simulink model "Cruise_Model_V8_QRTuning_LQI"  (R2024a)
settings: Solver=ode23t  StartTime=0.0  StopTime=20  RelTol=1e-3
values from neighbouring files (symbols this model uses):
  coefficients =     [UAM2.mat]    (also in VX4_cur.mat; VX4data.mat; alexisignoringme11UAM2.mat; alexisignoringme12.mat)
  Kpi = lqr(sys, Q, R)    [QRerr_LQI.m]    (also in alexisignoringme8.mat = [9.62344892608e-17 -1.21933000029e-16 1.4312558077e-15 29.45)
  mission =     [alexisignoringme.mat]    (also in alexisignoringme11UAM2.mat; alexisignoringme12.mat; alexisignoringme13.mat; alexisignoringme14.mat)
  q = 0.5*1.225*airflow.U^2    [VLMV3.m]    (also in VLMV3_modified.m = 0.5*1.225*airflow.U^2*Sref)
  referenceGeo =     [VX4data.mat]    (also in alexisignoringme.mat; alexisignoringme11UAM2.mat; alexisignoringme12.mat; alexisignoringme13.mat)
  Ue = U(:,idx(2)+1)    [QRerr_LQI.m]    (also in QRerr_p.m; alexisignoringme4.mat = [0.01662518914 6.61806403433e-08 9.21309449136e-07 1460.2523; alexisignoringme5.mat = [0 0 0 0 0 -1471.90874183 1.06985703496e-06 -4.11944256484e-; alexisignoringme6.mat = [0 0 0 0 0 -1471.90874183 1.06985703496e-06 -4.11944256484e-)
  X = [0.00351660116596 0 -9.99999602467 0 0 0 2.75026701025e-08 -4.1982332666e-06 -1.5333765693e-08 0.000503097278932 0 -6.54626389426e-11 ... (630 elements, 9x5x14)]    [alexisignoringme.mat]    (also in alexisignoringme12.mat = [0.000256495736971 0 -9.99999647184 0 0 0 0 -3.73764411116e-; alexisignoringme13.mat = [0.00833666803911 0 -10.0000021435 0 0 0 0 7.14203458163e-06; alexisignoringme14.mat = [0.00833666803911 0 -10.0000021435 0 0 0 0 7.14203458163e-06; alexisignoringme4.mat = [0.00351658839646 0 -9.99999599468 0 0 0 2.7327442949e-09 -4)
  Xe = X(:,idx(2)+1)    [QRerr_LQI.m]    (also in QRerr_p.m; alexisignoringme4.mat = [24.9726490597 0 -1.16896704065 0 0 0 -8.24889531393e-07 -0.; alexisignoringme5.mat = [24.9726490597 0 -1.16896704065 0 0 0 -8.24889531393e-07 0.0; alexisignoringme6.mat = [24.9726490597 0 -1.16896704065 0 0 0 -8.24889531393e-07 0.0)
  Xes = X(:,idx(2))    [QRerr_LQI.m]    (also in QRerr_p.m; alexisignoringme4.mat = [0.00351658839646 0 -9.99999599468 0 0 0 2.7327442949e-09 -4; alexisignoringme5.mat = [0 0 -1.11199998303 0 0 0 -1.38069247376e-09 1.48137256273e-; alexisignoringme6.mat = [0 0 -1.11199998303 0 0 0 -1.38069247376e-09 1.48137256273e-)
undefined symbols (not defined in the file or in its folder): F, Light, MIL
libraries: slpidlib x14, aerolibwind2 x8, aerolibatmos2 x4, shared6dof x1
(part 3 of 3)

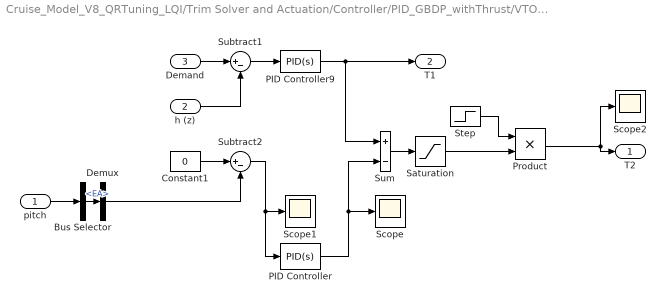
== system Cruise_Model_V8_QRTuning_LQI/Trim Solver and Actuation/Controller/PID_GBDP_withThrust/VTOL Control Path ==
  pitch : Inport
  h (z) : Inport  Port=2
  Demand : Inport  Port=3
  Bus Selector : BusSelector  OutputSignals=EA
  Constant1 : Constant  Value=0
  Demux : Demux  Outputs=3
  PID Controller : slpidlib/PID Controller  Controller=PID  Form=Parallel  TimeDomain=Continuous-time  UseExternalTs=off  SampleTime=-1  IntegratorMethod=Forward Euler  FilterMethod=Forward Euler  ControllerParametersSource=internal  P=2347  I=2604  UseKiTs=off  D=519  UseExternalDerivativeSource=off  N=129  UseFilter=on  TunerSelectOption=Transfer Function Based (PID Tuner App)  InitialConditionSource=internal  InitialConditionForIntegrator=0  InitialConditionForFilter=0  DifferentiatorICPrevScaledInput=0  ExternalReset=none  TrackingMode=off  Kt=1  LimitOutput=on  SatLimitsSource=internal  UpperSaturationLimit=800  LowerSaturationLimit=-800  LinearizeAsGain=on  AntiWindupMode=clamping  Kb=1  LimitIntegrator=off  UpperIntegratorSaturationLimit=inf  LowerIntegratorSaturationLimit=-inf  POutMin=[]  POutMax=[]  IOutMin=[]  IOutMax=[]  DOutMin=[]  DOutMax=[]  NOutMin=[]  NOutMax=[]  SumOutMin=[]  SumOutMax=[]  SaturationOutMin=[]  SaturationOutMax=[]  PParamMin=[]  PParamMax=[]  IParamMin=[]  IParamMax=[]  DParamMin=[]  DParamMax=[]  NParamMin=[]  NParamMax=[]  KbParamMin=[]  KbParamMax=[]  KtParamMin=[]  KtParamMax=[]  KbOutMin=[]  KbOutMax=[]  KtOutMin=[]  KtOutMax=[]  IntegratorOutMin=[]  IntegratorOutMax=[]  FilterOutMin=[]  FilterOutMax=[]  SumI1OutMin=[]  SumI1OutMax=[]  SumI2OutMin=[]  SumI2OutMax=[]  SumI3OutMin=[]  SumI3OutMax=[]  SumI4OutMin=[]  SumI4OutMax=[]  SumDOutMin=[]  SumDOutMax=[]  DifferentiatorOutMin=[]  DifferentiatorOutMax=[]  FilterDiffOutCoefMin=[]  FilterDiffOutCoefMax=[]  ReciprocalOutMin=[]  ReciprocalOutMax=[]  SumDenOutMin=[]  SumDenOutMax=[]  SumNumOutMin=[]  SumNumOutMax=[]  DivideOutMin=[]  DivideOutMax=[]  UdiffTsProdOutMin=[]  UdiffTsProdOutMax=[]  NTsProdOutMin=[]  NTsProdOutMax=[]  UintegralTsProdOutMin=[]  UintegralTsProdOutMax=[]  UngainTsProdOutMin=[]  UngainTsProdOutMax=[]  ClampingZeroOutDataTypeStr=Inherit: Inherit via back propagation  ClampingZeroOutMin=[]  ClampingZeroOutMax=[]  FilterDenConstantOutDataTypeStr=Inherit: Inherit via back propagation  FilterDenConstantOutMin=[]  FilterDenConstantOutMax=[]  PCopyOutDataTypeStr=Inherit: Inherit via back propagation  PCopyOutMin=[]  PCopyOutMax=[]  NCopyOutDataTypeStr=Inherit: Inherit via back propagation  NCopyOutMin=[]  NCopyOutMax=[]  IntegratorContinuousStateAttributes=''  IntegratorStateMustResolveToSignalObject=off  IntegratorRTWStateStorageClass=Auto  FilterContinuousStateAttributes=''  FilterStateMustResolveToSignalObject=off  FilterRTWStateStorageClass=Auto  ParallelPVariant=InternalParameters  IdealPVariant=Disabled  IVariant=InternalParameters  DVariant=InternalParameters  IntegratorVariant=Continuous  SatVariant=Enabled  AWVariant=ContClampingParallel  PCopyVariant=Disabled  TRVariant=Disabled  FdbkBlocksVariant=Forward  IdealPFdbkVariant=Disabled  SatFdbkVariant=Disabled  DerivativeFilterVariant=ContFilter  NVariant=InternalParameters  NCopyVariant=Disabled  FilterICVariant=InternalICsFilter  IntegratorICVariant=InternalICs  ExternalResetVariant=Disabled  TRSumVariant=Passthrough  SumFdbkVariant=Disabled  SumVariant=Sum_PID  TsampFilterVariant=InternalTs  TsampNgainVariant=Passthrough  TsampIntegralVariant=Disabled_SignalSpec  ExternalSaturationOutDataTypeStr=Inherit: Same as second input  DerivativeSourceVariant=ErrorSignal
  PID Controller9 : slpidlib/PID Controller  Controller=PID  Form=Parallel  TimeDomain=Continuous-time  UseExternalTs=off  SampleTime=-1  IntegratorMethod=Forward Euler  FilterMethod=Forward Euler  ControllerParametersSource=internal  P=-174.901958260333  I=-41.0371926298995  UseKiTs=off  D=-183.043785953636  UseExternalDerivativeSource=off  N=27.3346026399604  UseFilter=on  TunerSelectOption=Transfer Function Based (PID Tuner App)  InitialConditionSource=internal  InitialConditionForIntegrator=0  InitialConditionForFilter=0  DifferentiatorICPrevScaledInput=0  ExternalReset=none  TrackingMode=off  Kt=1  LimitOutput=on  SatLimitsSource=internal  UpperSaturationLimit=2000  LowerSaturationLimit=0  LinearizeAsGain=off  AntiWindupMode=clamping  Kb=1  LimitIntegrator=off  UpperIntegratorSaturationLimit=inf  LowerIntegratorSaturationLimit=-inf  POutMin=[]  POutMax=[]  IOutMin=[]  IOutMax=[]  DOutMin=[]  DOutMax=[]  NOutMin=[]  NOutMax=[]  SumOutMin=[]  SumOutMax=[]  SaturationOutMin=[]  SaturationOutMax=[]  PParamMin=[]  PParamMax=[]  IParamMin=[]  IParamMax=[]  DParamMin=[]  DParamMax=[]  NParamMin=[]  NParamMax=[]  KbParamMin=[]  KbParamMax=[]  KtParamMin=[]  KtParamMax=[]  KbOutMin=[]  KbOutMax=[]  KtOutMin=[]  KtOutMax=[]  IntegratorOutMin=[]  IntegratorOutMax=[]  FilterOutMin=[]  FilterOutMax=[]  SumI1OutMin=[]  SumI1OutMax=[]  SumI2OutMin=[]  SumI2OutMax=[]  SumI3OutMin=[]  SumI3OutMax=[]  SumI4OutMin=[]  SumI4OutMax=[]  SumDOutMin=[]  SumDOutMax=[]  DifferentiatorOutMin=[]  DifferentiatorOutMax=[]  FilterDiffOutCoefMin=[]  FilterDiffOutCoefMax=[]  ReciprocalOutMin=[]  ReciprocalOutMax=[]  SumDenOutMin=[]  SumDenOutMax=[]  SumNumOutMin=[]  SumNumOutMax=[]  DivideOutMin=[]  DivideOutMax=[]  UdiffTsProdOutMin=[]  UdiffTsProdOutMax=[]  NTsProdOutMin=[]  NTsProdOutMax=[]  UintegralTsProdOutMin=[]  UintegralTsProdOutMax=[]  UngainTsProdOutMin=[]  UngainTsProdOutMax=[]  ClampingZeroOutDataTypeStr=Inherit: Inherit via back propagation  ClampingZeroOutMin=[]  ClampingZeroOutMax=[]  FilterDenConstantOutDataTypeStr=Inherit: Inherit via back propagation  FilterDenConstantOutMin=[]  FilterDenConstantOutMax=[]  PCopyOutDataTypeStr=Inherit: Inherit via back propagation  PCopyOutMin=[]  PCopyOutMax=[]  NCopyOutDataTypeStr=Inherit: Inherit via back propagation  NCopyOutMin=[]  NCopyOutMax=[]  IntegratorContinuousStateAttributes=''  IntegratorStateMustResolveToSignalObject=off  IntegratorRTWStateStorageClass=Auto  FilterContinuousStateAttributes=''  FilterStateMustResolveToSignalObject=off  FilterRTWStateStorageClass=Auto  ParallelPVariant=InternalParameters  IdealPVariant=Disabled  IVariant=InternalParameters  DVariant=InternalParameters  IntegratorVariant=Continuous  SatVariant=Enabled  AWVariant=ContClampingParallel  PCopyVariant=Disabled  TRVariant=Disabled  FdbkBlocksVariant=Forward  IdealPFdbkVariant=Disabled  SatFdbkVariant=Disabled  DerivativeFilterVariant=ContFilter  NVariant=InternalParameters  NCopyVariant=Disabled  FilterICVariant=InternalICsFilter  IntegratorICVariant=InternalICs  ExternalResetVariant=Disabled  TRSumVariant=Passthrough  SumFdbkVariant=Disabled  SumVariant=Sum_PID  TsampFilterVariant=InternalTs  TsampNgainVariant=Passthrough  TsampIntegralVariant=Disabled_SignalSpec  ExternalSaturationOutDataTypeStr=Inherit: Same as second input  DerivativeSourceVariant=ErrorSignal
  Product : Product
  Saturation : Saturate  UpperLimit=9000  LowerLimit=0
  Scope : Scope
  Scope1 : Scope
  Scope2 : Scope
  Step : Step  Time=max(mission.trans.t)  Before=1  After=0  SampleTime=0
  Subtract1 : Sum  Inputs=|+-
  Subtract2 : Sum  Inputs=|+-
  Sum : Sum  Inputs=+-
  T2 : Outport
  T1 : Outport  Port=2
  wires:
  Demand/1 -> Subtract1/1
  h (z)/1 -> Subtract1/2
  Subtract1/1 -> PID Controller9/1
  Constant1/1 -> Subtract2/1
  pitch/1 -> Bus Selector/1
  Subtract2/1 -> PID Controller/1, Scope1/1
  PID Controller9/1 -> Sum/1, T1/1
  Sum/1 -> Saturation/1
  PID Controller/1 -> Sum/2, Scope/1
  Bus Selector/1 -> Demux/1  "<EA>"
  Demux/2 -> Subtract2/2
  Product/1 -> T2/1, Scope2/1
  Saturation/1 -> Product/2
  Step/1 -> Product/1

== system Cruise_Model_V8_QRTuning_LQI/Trim Solver and Actuation/Controller/Trim Solver/Saturation4 ==
  In1 : Inport
  Demux3 : Demux  Outputs=9
  Mux : Mux  Inputs=9
  Saturation : Saturate
  Saturation1 : Saturate
  Saturation2 : Saturate
  Saturation3 : Saturate  UpperLimit=0  LowerLimit=-1.6*150*9.81
  Saturation4 : Saturate  UpperLimit=0  LowerLimit=-1.6*150*9.81
  Saturation5 : Saturate  UpperLimit=0  LowerLimit=-1.6*150*9.81
  Saturation6 : Saturate  UpperLimit=700  LowerLimit=-700
  Saturation7 : Saturate  UpperLimit=700  LowerLimit=-700
  Saturation8 : Saturate  UpperLimit=700  LowerLimit=-700
  Out1 : Outport
  wires:
  In1/1 -> Demux3/1
  Mux/1 -> Out1/1
  Demux3/1 -> Saturation/1
  Saturation/1 -> Mux/1
  Saturation1/1 -> Mux/2
  Demux3/2 -> Saturation1/1
  Saturation2/1 -> Mux/3
  Demux3/3 -> Saturation2/1
  Demux3/4 -> Saturation3/1
  Saturation3/1 -> Mux/4
  Demux3/5 -> Saturation4/1
  Saturation4/1 -> Mux/5
  Saturation5/1 -> Mux/6
  Demux3/6 -> Saturation5/1
  Saturation6/1 -> Mux/7
  Demux3/7 -> Saturation6/1
  Saturation7/1 -> Mux/8
  Demux3/8 -> Saturation7/1
  Saturation8/1 -> Mux/9
  Demux3/9 -> Saturation8/1

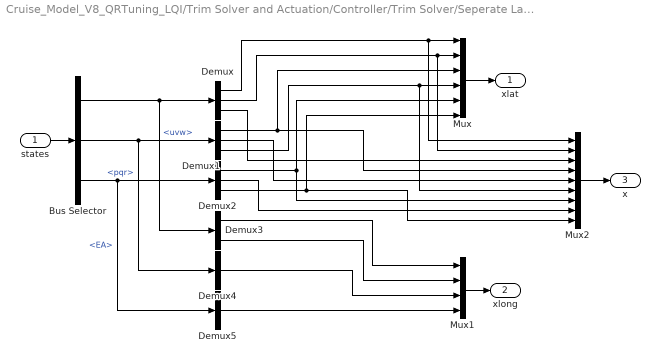
== system Cruise_Model_V8_QRTuning_LQI/Trim Solver and Actuation/Controller/Trim Solver/Seperate Lateral//Longitudinal ==
  states : Inport
  Bus Selector : BusSelector  OutputSignals=uvw,pqr,EA
  Demux{,1..5} (6 alike) : Demux  Outputs=3
  Mux : Mux  Inputs=6
  Mux1 : Mux
  Mux2 : Mux  Inputs=9
  xlat : Outport
  xlong : Outport  Port=2
  x : Outport  Port=3
  wires:
  states/1 -> Bus Selector/1
  Mux/1 -> xlat/1
  Mux1/1 -> xlong/1
  Bus Selector/1 -> Demux/1, Demux3/1  "<uvw>"
  Bus Selector/2 -> Demux1/1, Demux4/1  "<pqr>"
  Bus Selector/3 -> Demux5/1, Demux2/1  "<EA>"
  Demux/1 -> Mux2/1, Mux/1
  Demux/2 -> Mux2/2, Mux/2
  Demux1/1 -> Mux2/4, Mux/3
  Demux1/3 -> Mux2/6, Mux/4
  Demux2/1 -> Mux2/7, Mux/5
  Demux2/3 -> Mux2/9, Mux/6
  Demux3/1 -> Mux1/1
  Demux3/3 -> Mux1/2
  Demux4/2 -> Mux1/3
  Demux5/2 -> Mux1/4
  Mux2/1 -> x/1
  Demux/3 -> Mux2/3
  Demux1/2 -> Mux2/5
  Demux2/2 -> Mux2/8

== system Cruise_Model_V8_QRTuning_LQI/Trim Solver and Actuation/Controller/Trim Solver/Stop Time (Real) ==
  note: Source: Phillippe Martin (2016)
  note: https://www.researchgate.net/post/How-can-I-put-the-REAL-elapsed-time-as-a-constraint-in-a-Simulink-simulation
  Constant : Constant  Value=7
  Display : Display  Commented=on
  MATLAB Function : MATLAB Function  TreatAsAtomicUnit=on
  Relational Operator : RelationalOperator  OutDataTypeStr=boolean  InputSameDT=off
  Stop Simulation : Stop
  wires:
  Constant/1 -> Relational Operator/2
  Relational Operator/1 -> Stop Simulation/1
  MATLAB Function/1(y) -> Display/1, Relational Operator/1

== system Cruise_Model_V8_QRTuning_LQI/Trim Solver and Actuation/Controller/Trim Solver/Subsystem1 ==
  1-D Lookup Table : Lookup_n-D  NumberOfTableDimensions=1  BreakpointsForDimension1=[0 120]  Table=[X(1,1); X(1,20)]  InternalRulePriority=Speed  RndMeth=Simplest
  1-D Lookup Table1 : Lookup_n-D  NumberOfTableDimensions=1  BreakpointsForDimension1=[0 120]  Table=[X(2,1); X(2,20)]  InternalRulePriority=Speed  RndMeth=Simplest
  1-D Lookup Table2 : Lookup_n-D  NumberOfTableDimensions=1  BreakpointsForDimension1=[0 10 120]  Table=[X(3,1); X(3,1); X(3,20)]  InternalRulePriority=Speed  RndMeth=Simplest
  1-D Lookup Table3 : Lookup_n-D  NumberOfTableDimensions=1  BreakpointsForDimension1=[0 120]  Table=[X(4,1); X(4,20)]  InternalRulePriority=Speed  RndMeth=Simplest
  1-D Lookup Table4 : Lookup_n-D  NumberOfTableDimensions=1  BreakpointsForDimension1=[0 120]  Table=[X(5,1); X(5,20)]  InternalRulePriority=Speed  RndMeth=Simplest
  1-D Lookup Table5 : Lookup_n-D  NumberOfTableDimensions=1  BreakpointsForDimension1=[0 120]  Table=[X(6,1); X(6,20)]  InternalRulePriority=Speed  RndMeth=Simplest
  1-D Lookup Table6 : Lookup_n-D  NumberOfTableDimensions=1  BreakpointsForDimension1=[0 120]  Table=[X(7,1); X(7,20)]  InternalRulePriority=Speed  RndMeth=Simplest
  1-D Lookup Table7 : Lookup_n-D  NumberOfTableDimensions=1  BreakpointsForDimension1=[0 120]  Table=[X(8,1); X(8,20)]  InternalRulePriority=Speed  RndMeth=Simplest
  1-D Lookup Table8 : Lookup_n-D  NumberOfTableDimensions=1  BreakpointsForDimension1=[0 120]  Table=[X(9,1); X(9,20)]  InternalRulePriority=Speed  RndMeth=Simplest
  Clock1 : Clock
  Mux : Mux  Inputs=9
  Out1 : Outport
  wires:
  Clock1/1 -> 1-D Lookup Table8/1, 1-D Lookup Table7/1, 1-D Lookup Table6/1, 1-D Lookup Table5/1, 1-D Lookup Table4/1, 1-D Lookup Table3/1, 1-D Lookup Table2/1, 1-D Lookup Table1/1, 1-D Lookup Table/1
  Mux/1 -> Out1/1
  1-D Lookup Table6/1 -> Mux/7
  1-D Lookup Table1/1 -> Mux/2
  1-D Lookup Table4/1 -> Mux/5
  1-D Lookup Table2/1 -> Mux/3
  1-D Lookup Table7/1 -> Mux/8
  1-D Lookup Table8/1 -> Mux/9
  1-D Lookup Table3/1 -> Mux/4
  1-D Lookup Table5/1 -> Mux/6
  1-D Lookup Table/1 -> Mux/1

== system Cruise_Model_V8_QRTuning_LQI/Trim Solver and Actuation/Controller/PID_GBDP_withThrust/Altitude Control Path/Step demand for testing ==
  In1 : Inport
  Mux1 : Mux  Inputs=2
  Scope2 : Scope
  Scope4 : Scope
  Step1 : Step  Time=60  Before=-500  After=-490  SampleTime=0
  Step2 : Step  Time=80  After=-10  SampleTime=0
  Step3 : Step  Time=120  After=20  SampleTime=0
  Step4 : Step  Time=120  After=20  SampleTime=0
  Sum : Sum  Inputs=++++
  To Workspace : ToWorkspace  VariableName=altitudeResponse  SaveFormat=Timeseries  SampleTime=-1
  Out1 : Outport
  wires:
  Step3/1 -> Sum/3
  Mux1/1 -> To Workspace/1, Scope4/1
  Sum/1 -> Out1/1, Mux1/1
  Step4/1 -> Sum/4
  Step1/1 -> Sum/1
  In1/1 -> Mux1/2, Scope2/1
  Step2/1 -> Sum/2

== system Cruise_Model_V8_QRTuning_LQI/Trim Solver and Actuation/Controller/PID_GBDP_withThrust/Course Angle Control Path/Step demand for testing2 ==
  Va : Inport
  Mux1 : Mux  Inputs=2
  Scope2 : Scope
  Scope4 : Scope
  Step1 : Step  Time=60  Before=0.1  After=0.2  SampleTime=0
  Step2 : Step  Time=80  After=-0.4  SampleTime=0
  Step3 : Step  Time=120  After=-0.2  SampleTime=0
  Step4 : Step  Time=100  After=0.6  SampleTime=0
  Step5 : Step  Time=140  After=-0.4  SampleTime=0
  Sum : Sum  Inputs=+++++
  To Workspace : ToWorkspace  VariableName=headingAngleResponse  SaveFormat=Timeseries  SampleTime=-1
  Out1 : Outport
  wires:
  Step5/1 -> Sum/5
  Step3/1 -> Sum/3
  Mux1/1 -> To Workspace/1, Scope4/1
  Sum/1 -> Out1/1, Mux1/1
  Step4/1 -> Sum/4
  Step1/1 -> Sum/1
  Va/1 -> Mux1/2, Scope2/1
  Step2/1 -> Sum/2

== system Cruise_Model_V8_QRTuning_LQI/Trim Solver and Actuation/Controller/PID_GBDP_withThrust/Subsystem/Step demand for testing1 ==
  Va : Inport
  Mux1 : Mux  Inputs=2
  Scope2 : Scope
  Scope4 : Scope
  Step1 : Step  Time=60  Before=25  After=31  SampleTime=0
  Step2 : Step  Time=80  After=-3  SampleTime=0
  Step3 : Step  Time=120  After=-5  SampleTime=0
  Step4 : Step  Time=100  After=8  SampleTime=0
  Step5 : Step  Time=140  After=-2  SampleTime=0
  Sum : Sum  Inputs=+++++
  To Workspace : ToWorkspace  VariableName=airspeedResponse  SaveFormat=Timeseries  SampleTime=-1
  Out1 : Outport
  wires:
  Step2/1 -> Sum/2
  Va/1 -> Scope2/1, Mux1/2
  Step1/1 -> Sum/1
  Step4/1 -> Sum/4
  Sum/1 -> Mux1/1, Out1/1
  Mux1/1 -> Scope4/1, To Workspace/1
  Step3/1 -> Sum/3
  Step5/1 -> Sum/5

== matlab function Cruise_Model_V8_QRTuning_LQI/Trim Solver and Actuation/Controller/Trim Solver/Stop Time (Real)/MATLAB Function ==
  data: y output
function y = fcn()
%#codegen

persistent t0
coder.extrinsic('cputime');

if isempty(t0)
    y = 0;
    t0 = 0;
    t0 = cputime;
end

y = cputime;
y = y-t0;

== matlab function Cruise_Model_V8_QRTuning_LQI/Aircraft Dynamics/Aerodynamic Forces and Moments/MATLAB Function ==
  data: Fb output; Mcg output; coeff input Bus: coeff; u input; alpha input; beta input; V input; rho input; X input; refGeo parameter; m parameter; thrust input; cg parameter
function [Fb,Mcg] = aeroDyn(coeff, u, alpha, beta, V, rho, X, refGeo, m, thrust, cg)
% Function aeroDyn simulates ....

%% Setting up intermediate variables
b = refGeo.bref;
S = refGeo.Sref;
c = refGeo.cref;

Q = 0.5*rho*V^2; % Dynamic pressure Q

ndc = c/(2*V);
ndb = b/(2*V);

%% Seperating vectors (BFR)
uvw = X(1:3); % Translational velocity vector
pqr = X(4:6); % Angular velocity vector
EA = X(7:end);

%% Handle Stall

%% Non-dimensional Aerodynamic Force Coefficients
% In wind axis
% Lift
CL = applyDeriv(coeff.CL0, coeff.CLa, coeff.CLb, coeff.CLn, 0, coeff.CLq, 0, u, alpha, beta, pqr, ndc);

% Drag 
CD = applyDeriv(coeff.CD0, coeff.CDa, coeff.CDb, coeff.CDn, 0, 0, 0, u, alpha, beta, pqr, ndc);

% Sideforce
CY = applyDeriv(0, coeff.CYa, coeff.CYb, coeff.CYn, coeff.CYp, 0, coeff.CYr, u, alpha, beta, pqr, ndb);

if abs(alpha) > 14.5*(pi/180)
    CL = 0;
    CD = coeff.CD0;
    CY = 0;
end

%% Rotate wind to body
Faw = [-max(CD,0); CY; -CL].*Q*S; % Force vector in the stability frame

Rwb = [cos(alpha)*cos(beta), -cos(alpha)*sin(beta), -sin(alpha);  
       sin(beta)           ,  cos(beta)           ,  0         ; 
       cos(beta)*sin(alpha), -sin(alpha)*sin(beta),  cos(alpha)];

Fab = Rwb*Faw; % aerodynamic force on body

%% Aerodynamic Moment about CG
% In Fb, with moments taken about the centre of gravity

% Roll
Cl = applyDeriv(0, coeff.Cla, coeff.Clb, coeff.Cln, coeff.Clp, 0, coeff.Clr, u, alpha, beta, pqr, ndb);

% Pitch
Cm = applyDeriv(coeff.Cm0, coeff.Cma, coeff.Cmb, coeff.Cmn, 0, coeff.Cmq, 0, u, alpha, beta, pqr, ndc);

% Yaw
Cn = applyDeriv(0, coeff.Cna, coeff.Cnb, coeff.Cnn, coeff.Cnp, 0, coeff.Cnr, u, alpha, beta, pqr, ndb);

if abs(alpha) > 20*(pi/180)
    Cm = 0;
    Cn = 0;
    Cl = 0;
end

Ma = [b*Cl; c*Cm; b*Cn].*Q*S;

%% Propulsion Effects
% Moment and forces induced by throttle
FTb = u(4:6);
MTcg = u(7:9);

% Gravity Effects
Fgb = [-9.81*sin(X(8))          ; % Body frame
        9.81*cos(X(8))*sin(X(7));
        9.81*cos(X(8))*cos(X(7))]*m; % ASSUMPTION: Constant Mass

%% Out
Rbe = body2earth(X(7), X(8), X(9));

Fb = FTb + Fgb + Fab;
Mcg = MTcg + Ma;

forces = [FTb; Fgb; Fab; Rbe*Fb];
aero = [CL; CD; Cm];
uvw_e = Rbe*X(1:3);

end

%% Extra functions

function C = applyDeriv(C0, Ca, Cb, Cn, Cp, Cq, Cr, u, alpha, beta, pqr, nd)
% function applyDeriv calculates the coefficient C from the derivatives C0,
% Ca, Cb, Cn wrt 0, alpha, beta and control (n), respectively.

    C_nc = C0 + Ca*alpha + Cb*beta + Cp*pqr(1)*nd + Cq*pqr(2)*nd + Cr*pqr(3)*nd; % lift coefficient no control
    
    C_c = (Cn.*u(1:length(Cn)))';

    C = C_nc + sum(C_c);

end
